simulink model "environment_subsystem"  (R2024a)
settings: Solver=VariableStepAuto  StartTime=0.0  StopTime=10.0  RelTol=1e-3
undefined symbols (not defined in the file): AUV
settings Model: Creator=adity  LastModifiedBy=adity

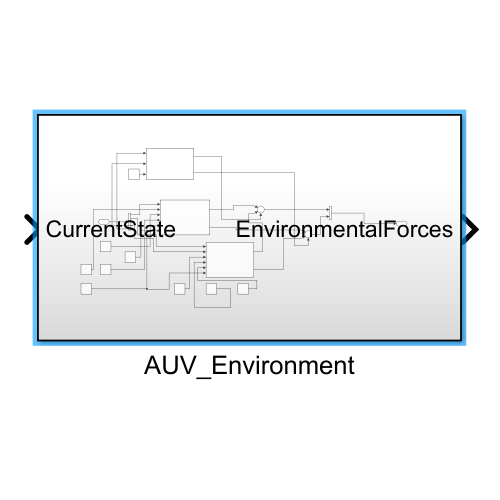
[thumbnail: Simulink's stored preview of the top-level diagram]
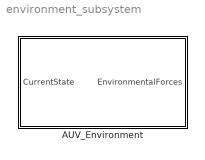
== system environment_subsystem ==
  AUV_Environment : Subsystem

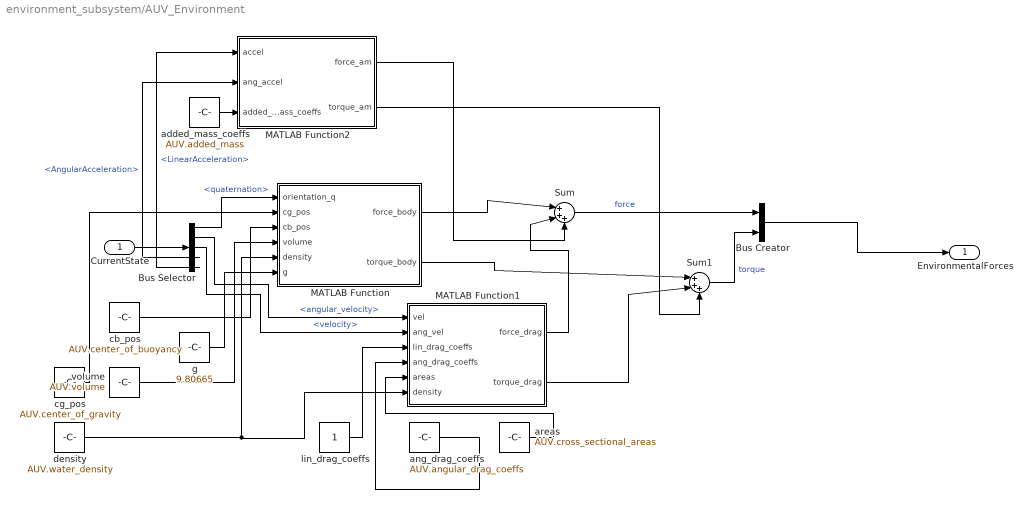
== system environment_subsystem/AUV_Environment ==
  CurrentState : Inport
  Bus Creator : BusCreator  Inputs=2
  Bus Selector : BusSelector  OutputSignals=quaternation,angular_velocity,velocity,AngularAcceleration,LinearAcceleration
  MATLAB Function : MATLAB Function  TreatAsAtomicUnit=on
  MATLAB Function1 : MATLAB Function  TreatAsAtomicUnit=on
  MATLAB Function2 : MATLAB Function  TreatAsAtomicUnit=on
  Sum : Sum  Inputs=|+++
  Sum1 : Sum  Inputs=|+++
  added_mass_coeffs : Constant  Value=AUV.added_mass
  ang_drag_coeffs : Constant  Value=AUV.angular_drag_coeffs
  areas : Constant  Value=AUV.cross_sectional_areas
  cb_pos : Constant  Value=AUV.center_of_buoyancy
  cg_pos : Constant  Value=AUV.center_of_gravity
  density : Constant  Value=AUV.water_density
  g : Constant  Value=9.80665
  lin_drag_coeffs : Constant
  volume : Constant  Value=AUV.volume
  EnvironmentalForces : Outport
  wires:
  CurrentState/1 -> Bus Selector/1
  Bus Selector/1 -> MATLAB Function/1(orientation_q)  "<quaternation>"
  cg_pos/1 -> MATLAB Function/2(cg_pos)
  cb_pos/1 -> MATLAB Function/3(cb_pos)
  volume/1 -> MATLAB Function/4(volume)
  density/1 -> MATLAB Function/5(density), MATLAB Function1/6(density)
  g/1 -> MATLAB Function/6(g)
  Bus Selector/2 -> MATLAB Function1/1(vel)  "<angular_velocity>"
  Bus Selector/3 -> MATLAB Function1/2(ang_vel)  "<velocity>"
  areas/1 -> MATLAB Function1/5(areas)
  ang_drag_coeffs/1 -> MATLAB Function1/4(ang_drag_coeffs)
  lin_drag_coeffs/1 -> MATLAB Function1/3(lin_drag_coeffs)
  MATLAB Function/1(force_body) -> Sum/1
  MATLAB Function1/1(force_drag) -> Sum/2
  MATLAB Function/2(torque_body) -> Sum1/1
  MATLAB Function1/2(torque_drag) -> Sum1/2
  Sum/1 -> Bus Creator/1  "force"
  Sum1/1 -> Bus Creator/2  "torque"
  Bus Creator/1 -> EnvironmentalForces/1
  Bus Selector/4 -> MATLAB Function2/2(ang_accel)  "<AngularAcceleration>"
  Bus Selector/5 -> MATLAB Function2/1(accel)  "<LinearAcceleration>"
  added_mass_coeffs/1 -> MATLAB Function2/3(added_mass_coeffs)
  MATLAB Function2/2(torque_am) -> Sum1/3
  MATLAB Function2/1(force_am) -> Sum/3

== matlab function environment_subsystem/AUV_Environment/MATLAB Function1 ==
  data: vel input; force_drag output; ang_vel input; lin_drag_coeffs input; ang_drag_coeffs input; areas input; density input; torque_drag output
function [force_drag, torque_drag] = drag_model(vel, ang_vel, lin_drag_coeffs, ang_drag_coeffs, areas, density)
    % Calculates hydrodynamic drag forces and torques in the body frame
    % vel:      Linear velocity vector [vx, vy, vz]
    % ang_vel:  Angular velocity vector [p, q, r]

    % --- Linear Drag ---
    % Using the quadratic drag formula: Fd = -0.5 * rho * v^2 * Cd * A
    % The sign() function ensures the force always opposes the velocity.
    force_drag = -sign(vel) .* (0.5 * density .* (vel.^2) .* lin_drag_coeffs .* areas);

    % --- Angular Drag (Rotational Resistance) ---
    % A similar model for rotational drag. We use a length^5 term for scaling,
    % assuming a characteristic length of 1m for simplicity.
    torque_drag = -sign(ang_vel) .* (0.5 * density .* (ang_vel.^2) .* ang_drag_coeffs);
endfunction y = fcn(u)

y = u;

== matlab function environment_subsystem/AUV_Environment/MATLAB Function ==
  data: orientation_q input; force_body output; cg_pos input; cb_pos input; volume input; density input; g input; torque_body output
function [force_body, torque_body] = buoyancy_model(orientation_q, cg_pos, cb_pos, volume, density, g)
    % This function calculates buoyancy force and torque in the AUV's body frame.
    % orientation_q: quaternion [w, x, y, z] from the plant
    % cg_pos: Center of Gravity position vector [x, y, z] in body frame
    % cb_pos: Center of Buoyancy position vector [x, y, z] in body frame

    % 1. Calculate the buoyant force vector in the world frame (upward)
    force_magnitude = volume * density * g;
    force_world = [0; 0; -force_magnitude]; % Upward force in our Z-down world

    % 2. Rotate the world force vector into the AUV's body frame
    % We use the inverse of the AUV's orientation to rotate a world vector to body
    force_body = quatrotate(quatinv(orientation_q), force_world')';

    % 3. Calculate the torque produced by this force acting at the Center of Buoyancy
    % Torque = r x F, where r is the vector from the CG to the CB
    lever_arm = cb_pos - cg_pos;
    torque_body = cross(lever_arm, force_body);
end

== matlab function environment_subsystem/AUV_Environment/MATLAB Function2 ==
  data: accel input; force_am output; ang_accel input; added_mass_coeffs input; torque_am output
function [force_am, torque_am] = added_mass_model(accel, ang_accel, added_mass_coeffs)
    % Calculates the forces and torques due to added mass.
    % F = -m_added * acceleration

    % Split the 6-element coeff vector into linear and angular parts
    added_mass_linear = added_mass_coeffs(1:3);
    added_mass_angular = added_mass_coeffs(4:6);

    force_am = -added_mass_linear .* accel;
    torque_am = -added_mass_angular .* ang_accel;
end
